simulink model "sldemo_fuelsys_original"  (R2017a)
settings: Solver=FixedStepAuto  StartTime=0  StopTime=30  FixedStep=0.001  RelTol=1e-5  AbsTol=1e-6
PostLoadFcn:
  | sldemo_fuelsys_data(bdroot,'initialize_data','orig','float');
model workspace (MAT data in the model file):
  PressEst = [0.806253176324 0.553142316929 0.37151500209 0.277667903103 0.220198954207 0.181288665766 0.153200000489 0.115431020872 0.0913067476324 0.0746519188607 0.0625231108324 0.0533383634277 ... (306 elements, 18x17)]
  PressVect = [0.05 0.1 0.15 0.2 0.25 0.3 0.35 0.4 0.45 0.5 0.55 0.6 ... (19 elements, 1x19)]
  PumpCon = [-0.0556348 -0.0022828 0.0256932 0.0435188 0.0562692 0.0661194857143 0.0741572 0.08697 0.0972452 0.106070342857 0.1139892 0.121303866667 ... (342 elements, 18x19)]
  RampRateKiX = [100 200 300 400 500 600]
  RampRateKiY = [0 0.2 0.4 0.6 0.8 1]
  RampRateKiZ = [0.012 0.024 0.036 0.048 0.06 0.072 0.024 0.048 0.072 0.096 0.12 0.144 ... (36 elements, 6x6)]
  SpeedEst = [471.837839721 550.80940091 777.559313277 1080.9243499 1418.36795322 1769.7468768 2125.37309264 2480.20345067 2831.37796793 3177.14006959 3516.32917143 4064.90417867 ... (323 elements, 17x19)]
  SpeedVect = [50 75 100 125 150 175 200 250 300 350 400 450 ... (18 elements, 1x18)]
  ThrotEst = [0 0 0 0 0 0 0 0 0 0 0 0 ... (342 elements, 18x19)]
  ThrotVect = [0 3 6 9 12 15 18 21 24 27 30 35 ... (17 elements, 1x17)]
  ego_sw = 1
  engine_speed = 300
  hys = 25
  map_sw = 1
  max_ego = 1.2
  max_press = 0.95
  max_speed = 628
  max_throt = 90
  min_press = 0.05
  min_speed = 50
  min_throt = 3
  speed_sw = 1
  st_range = 0.0001
  throttle_sw = 1
  zero_thresh = 250
undefined symbols (not defined in the file or in its folder): DiscIntNeverNeededParam, sld_FuelModes, sldvsubsys
libraries: simulink x3, simulink_extras x1
(part 2 of 2)

== matlab function sldemo_fuelsys_original/Engine_Gas_Dynamics/Throttle & Manifold/Throttle/f(theta) ==
  data: u input; y output
function y = f(u)
%#codegen

y = 2.821 - 0.05231*u + 0.10299*u^2 - 0.00063*u^3;

== matlab function sldemo_fuelsys_original/Engine_Gas_Dynamics/Throttle & Manifold/Throttle/g(pratio) ==
  data: u input; y output
function y = g(u)
%#codegen

y = 2*sqrt(abs(u - u^2));

== matlab function sldemo_fuelsys_original/Engine_Gas_Dynamics/Throttle & Manifold/Intake Manifold/MATLAB Function ==
  data: u1 input; y output; u2 input
function y = pumping(u1,u2)
%#codegen

y = -0.366 + 0.08979*u1*u2 - 0.0337*u2*u1^2 + 0.0001*u1*u2^2;

== matlab function sldemo_fuelsys_original/Engine_Gas_Dynamics/Mixing & Combustion/EGO Sensor ==
  data: u input; y output
function y = fcn(u)
%#codegen

y = (1-tanh(4*(u-14.6)))/2;
